simulink model "StandaloneDAQv07_R2014a"  (R2014a)
settings: Solver=FixedStepDiscrete  SolverMode=MultiTasking  StartTime=0.0  StopTime=inf  FixedStep=0.0005  RelTol=1e-3
values from neighbouring files (symbols this model uses):
  ANOMALY_INIT = 10    [DAQParams3_1ms_DDA.m]
  Calibration = getCalibrationParams_ATRIAS()    [DAQParams3_1ms_DDA.m]
  EnableFT = 0    [DAQParams3_1ms_DDA.m]
  EncoderAngleLimits = [60 240; 120 300; 60 240; 120 300; 60 240; 120 300; 60 240; 120 300; -30 30; -30 30; -inf inf; -inf inf; -inf inf; -inf inf; -30 30; -30 30; -inf inf; -90 90; -90 90]*pi/180    [DAQParams3_1ms_DDA.m]
  EncoderFiltSys = getDerivFilter(2, 5, 5, Ts)    [DAQParams3_1ms_DDA.m]
  EncoderThreshold = [5; 5; 5; 5; 5; 5; 5; 5; 5; 5; 250; 250; 250; 250; 5; 5; 5; 5; 5]*pi/180    [DAQParams3_1ms_DDA.m]
  IMUAngleLimits = [-180 180; -90 90; -90 90]*pi/180    [DAQParams3_1ms_DDA.m]
  IMUCommand = 70    [DAQParams3_1ms_DDA.m]
  IMUThreshold = 5*pi/180    (= 0.0872664625997)    [DAQParams3_1ms_DDA.m]
  MAX_ANOMALY = 30    [DAQParams3_1ms_DDA.m]
  MedullaCommand = 0    [DAQParams3_1ms_DDA.m]
  MicrostrainFiltSys = getDerivFilter(2, 5, 5, TsMicrostrain)    [DAQParams3_1ms_DDA.m]
  MODBUS_TIMEOUT = 0.02    [DAQParams3_1ms_DDA.m]
  ResetDAQ = 0    [DAQParams3_1ms_DDA.m]
  ResetYaw = 0    [DAQParams3_1ms_DDA.m]
  STREAMING_TIMEOUT = 0.1    [DAQParams3_1ms_DDA.m]
  TareFT = 0    [DAQParams3_1ms_DDA.m]
  Ts = 0.001    [DAQParams3_1ms_DDA.m]
  UseMicrostrainRate = 0    [DAQParams3_1ms_DDA.m]
undefined symbols (not defined in the file or in its folder): FTCalibration, GearOffset, IMUTorsoOffset, m_XR17D15x, standard
libraries: xpcethercatlib x167, speedgoatlib x13, dspswit3 x2, simulink x2, xpcseriallib x1, SpeedgoatModified x1
(part 3 of 4)

== matlab function StandaloneDAQv07_R2014a/EtherCATNetwork/ComputeEulerAngles ==
  data: RkIn input; wk input; RCal input; Reset input; R0In input; ZYX output; dZYX output; Rk output; R0 output; YawRolloverIn input; YawRollover output
function [ZYX, dZYX, Rk, R0, YawRollover] = fcn(RkIn, wk, RCal, Reset, R0In, YawRolloverIn) %#codegen
    % Convert from IMU frame to robot frame and compute Euler angles. The
    % yaw angle is zeroed whenever (Reset) is true.
        
    if (Reset)
        % Compute the rotation matrix which zeroes the initial yaw
        qT0 = M_to_ZYX(RkIn*RCal);
        R0  = Rz(-qT0(1));
    else
        R0 = R0In;
    end
    
    % Transform from IMU to robot frame and zero initial yaw
    Rk = R0*RkIn*RCal;
    
    % Convert Rk to ZYX Euler angles
    ZYX = M_to_ZYX(Rk);
    
    % Unroll yaw
    YawRolloverCount = YawRolloverIn(1);
    PreviousYaw      = YawRolloverIn(2);
    CurrentYaw       = ZYX(1);
    YawRolloverCount = YawRolloverCount + getYawRollover(CurrentYaw, PreviousYaw);
    YawRollover      = [YawRolloverCount; CurrentYaw];
    ZYX(1)           = ZYX(1) + 2*pi*YawRolloverCount;
    
    % Compute Euler angle derivatives
    qzT = ZYX(1);
    qyT = ZYX(2);
    
    if cos(qyT)>1e-3
        dZYX = [0 -sin(qzT) cos(qzT)*cos(qyT); 0 cos(qzT) sin(qzT)*cos(qyT); 1 0 -sin(qyT)]\(R0*RkIn*wk);
    else
        dZYX = [0; 0; 0];
    end
end

function R = Rz(t)
    R = [cos(t) -sin(t) 0; sin(t) cos(t) 0; 0 0 1];
end

function Rollover = getYawRollover(CurrentYaw, PreviousYaw)
    % Determine if a rollover has occurred on yaw angle If a rollover is
    % detected, the output Rollover is either +1 or -1, depending on the
    % direction of the rollover.
  
    if (PreviousYaw>0 && CurrentYaw < (PreviousYaw-pi))
        Rollover = 1;
    elseif (PreviousYaw<0 && CurrentYaw > (PreviousYaw+pi))
        Rollover = -1;
    else
        Rollover = 0;
    end
end

== matlab function StandaloneDAQv07_R2014a/EtherCATNetwork/EtherCATRobotMicrostrain/ConvertAmpCurrent ==
  data: adc_value input; measuredCurrent output
function measuredCurrent = convert(adc_value)
    %#codegen

    measuredCurrent = (adc_value) * 60.0 / 8192;
end

== matlab function StandaloneDAQv07_R2014a/EtherCATNetwork/EtherCATRobotMicrostrain/ConvertLogicVoltage ==
  data: adc_value input; logicVoltage output
function logicVoltage = convert(adc_value)
    %#codegen
    
    MEDULLA_ADC_MAX_VOLTS     = 2.70;
    MEDULLA_ADC_OFFSET_COUNTS = 172;
    
    logicVoltage = (adc_value - MEDULLA_ADC_OFFSET_COUNTS) * (MEDULLA_ADC_MAX_VOLTS/(4095.0))  * 6.0;
end

== matlab function StandaloneDAQv07_R2014a/EtherCATNetwork/EtherCATRobotMicrostrain/ConvertThermistors ==
  data: Temperatures output; adc_value input
function Temperatures  = convert(adc_value)
    %#codegen
    MEDULLA_ADC_MAX_VOLTS     = 2.70;
    MEDULLA_ADC_OFFSET_COUNTS = 172;
    
    processedADCValue = (adc_value - MEDULLA_ADC_OFFSET_COUNTS) * (MEDULLA_ADC_MAX_VOLTS/(4095.0));
    Temperatures      = (1.0./( (1.0/298.15) + (1.0/3988.0)*log(4700.0./((3.26./processedADCValue) - 1.0)/10000))) - 273.15;
end

== matlab function StandaloneDAQv07_R2014a/StateEstimator/GeneralizedCoordinates ==
  data: EncoderAngles input; EncoderVelocities input; q_clean output; IMUAngles input; IMUVelocities input; UseMotorIncEncoders input; UseIMU input; dq_clean output; IMUTorsoOffset input; GearOffset input; Reset input
function [q_clean, dq_clean] = coords(EncoderAngles, EncoderVelocities, IMUAngles, IMUVelocities, UseMotorIncEncoders, UseIMU, IMUTorsoOffset, GearOffset, Reset)
    %#codegen
    
    % q_clean =
    %  [qzT; qyT; qxT; q1R; q2R; q1L; q2L; qgr1R; qgr2R; q3R; qgr1L; qgr2L; q3L];
    %
    % EncoderAngles = 
    %  [Leg1R; Leg2R; Leg1L; Leg2L; Motor1R; Motor2R; Motor1L; Motor2L; Hip3R; Hip3L; ...   % ABSOLUTE ENCODERS
    %   Inc1R; Inc2R; Inc1L; Inc2L; Inc3R; Inc3L; Boom; Boom; Boom]                         % INCREMENTAL ENCODERS
    
    if (Reset)
        q_clean  = zeros(13,1);
        dq_clean = zeros(13,1);
    else 
        q_clean  = EncoderAngles([17:19 1:6 15 7:8 16]);
        dq_clean = EncoderVelocities([17:19 1:6 15 7:8 16]);
        
        q_clean([8:9 11:12]) = q_clean([8:9 11:12]) + GearOffset*pi/180;
        if (UseMotorIncEncoders)
            if 0
                q_clean([8:9 11:12])  = EncoderAngles(11:14)/50;
                dq_clean([8:9 11:12]) = EncoderVelocities(11:14)/50;
            else
                % BGB 2014-08-29
                % The incremental encoder on q1L was destroyed in the 60V
                % power fault event, so it cannot be used until it is
                % replaced.
                q_clean([8:9 12])  = EncoderAngles([11:12 14])/50;
                dq_clean([8:9 12]) = EncoderVelocities([11:12 14])/50;
            end
        end
        
        if (UseIMU)
            q_clean(1:3)  = IMUAngles + [0; IMUTorsoOffset]*pi/180;
            dq_clean(1:3) = IMUVelocities;
        end
    end
end

== matlab function StandaloneDAQv07_R2014a/EtherCATNetwork/calibrate ==
  data: Calibration input; AbsEncoders input; IncEncoders input; IncEncodersPrev input; AbsAngle output; Reset input; IncAngle output; RolloverIn input; Rollover output; IncCalTickIn input; IncCalTick output
function [AbsAngle, IncAngle, Rollover, IncCalTick] = calibrate(Calibration,AbsEncoders,IncEncoders,IncEncodersPrev,Reset,RolloverIn,IncCalTickIn)
    %#codegen
    [AbsAngle, IncAngle, Rollover, IncCalTick] = calibrateEncoders2(Calibration,AbsEncoders,IncEncoders,IncEncodersPrev,Reset,RolloverIn,IncCalTickIn);
end

== matlab function StandaloneDAQv07_R2014a/EtherCATNetwork/EtherCATRobotMicrostrain/IMU_Medulla/TypecastAndCast ==
  data: u input uint32; y output
function y = unit32_to_double(u)
    %#codegen
    ys = typecast(u, 'single');
    y  = double(ys);
end

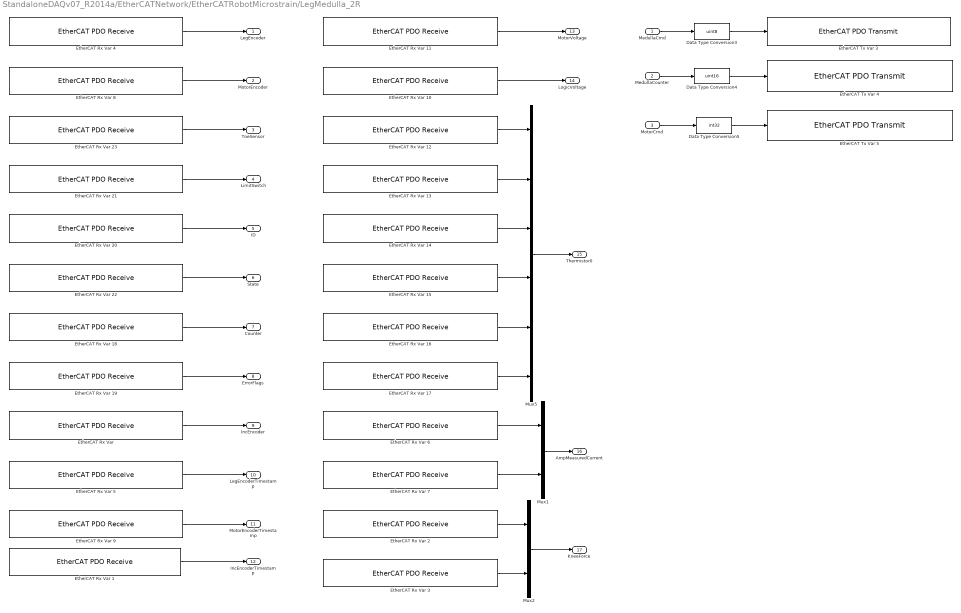
== system StandaloneDAQv07_R2014a/EtherCATNetwork/EtherCATRobotMicrostrain/LegMedulla_2R ==
  MedullaCmd : Inport
  MedullaCounter : Inport  Port=2
  MotorCmd : Inport  Port=3
  Data Type Conversion3 : DataTypeConversion  OutDataTypeStr=uint8  RndMeth=Simplest
  Data Type Conversion4 : DataTypeConversion  OutDataTypeStr=uint16  RndMeth=Simplest
  Data Type Conversion5 : DataTypeConversion  OutDataTypeStr=int32  RndMeth=Simplest
  "EtherCAT Rx Var " : xpcethercatlib/EtherCAT PDO Receive  Priority=2  sig_name=Box 4 (ATRIAS 2.1 Leg (Medulla 1.5)).Incremental Encoder.Incremental Encoder  sig_offset=1872  sig_type=uint16  type_size=16  sig_dim=1  device_id=0  sample_time=0.000500
  EtherCAT Rx Var 1 : xpcethercatlib/EtherCAT PDO Receive  Priority=2  sig_name=Box 4 (ATRIAS 2.1 Leg (Medulla 1.5)).Incremental Encoder.Incremental Encoder Timestamp  sig_offset=1888  sig_type=uint16  type_size=16  sig_dim=1  device_id=0  sample_time=0.000500
  EtherCAT Rx Var 10 : xpcethercatlib/EtherCAT PDO Receive  Priority=2  sig_name=Box 4 (ATRIAS 2.1 Leg (Medulla 1.5)).Power.Logic Voltage  sig_offset=1920  sig_type=uint16  type_size=16  sig_dim=1  device_id=0  sample_time=0.000500
  EtherCAT Rx Var 11 : xpcethercatlib/EtherCAT PDO Receive  Priority=2  sig_name=Box 4 (ATRIAS 2.1 Leg (Medulla 1.5)).Power.Motor Voltage  sig_offset=1904  sig_type=uint16  type_size=16  sig_dim=1  device_id=0  sample_time=0.000500
  EtherCAT Rx Var 12 : xpcethercatlib/EtherCAT PDO Receive  Priority=2  sig_name=Box 4 (ATRIAS 2.1 Leg (Medulla 1.5)).Thermistors.Thermistor 0  sig_offset=1936  sig_type=uint16  type_size=16  sig_dim=1  device_id=0  sample_time=0.000500
  EtherCAT Rx Var 13 : xpcethercatlib/EtherCAT PDO Receive  Priority=2  sig_name=Box 4 (ATRIAS 2.1 Leg (Medulla 1.5)).Thermistors.Thermistor 1  sig_offset=1952  sig_type=uint16  type_size=16  sig_dim=1  device_id=0  sample_time=0.000500
  EtherCAT Rx Var 14 : xpcethercatlib/EtherCAT PDO Receive  Priority=2  sig_name=Box 4 (ATRIAS 2.1 Leg (Medulla 1.5)).Thermistors.Thermistor 2  sig_offset=1968  sig_type=uint16  type_size=16  sig_dim=1  device_id=0  sample_time=0.000500
  EtherCAT Rx Var 15 : xpcethercatlib/EtherCAT PDO Receive  Priority=2  sig_name=Box 4 (ATRIAS 2.1 Leg (Medulla 1.5)).Thermistors.Thermistor 3  sig_offset=1984  sig_type=uint16  type_size=16  sig_dim=1  device_id=0  sample_time=0.000500
  EtherCAT Rx Var 16 : xpcethercatlib/EtherCAT PDO Receive  Priority=2  sig_name=Box 4 (ATRIAS 2.1 Leg (Medulla 1.5)).Thermistors.Thermistor 4  sig_offset=2000  sig_type=uint16  type_size=16  sig_dim=1  device_id=0  sample_time=0.000500
  EtherCAT Rx Var 17 : xpcethercatlib/EtherCAT PDO Receive  Priority=2  sig_name=Box 4 (ATRIAS 2.1 Leg (Medulla 1.5)).Thermistors.Thermistor 5  sig_offset=2016  sig_type=uint16  type_size=16  sig_dim=1  device_id=0  sample_time=0.000500
  EtherCAT Rx Var 18 : xpcethercatlib/EtherCAT PDO Receive  Priority=2  sig_name=Box 4 (ATRIAS 2.1 Leg (Medulla 1.5)).uController Status.Counter  sig_offset=1736  sig_type=uint8  type_size=8  sig_dim=1  device_id=0  sample_time=0.000500
  EtherCAT Rx Var 19 : xpcethercatlib/EtherCAT PDO Receive  Priority=2  sig_name=Box 4 (ATRIAS 2.1 Leg (Medulla 1.5)).uController Status.Error Flags  sig_offset=1744  sig_type=uint8  type_size=8  sig_dim=1  device_id=0  sample_time=0.000500
  EtherCAT Rx Var 2 : xpcethercatlib/EtherCAT PDO Receive  Priority=2  sig_name=Box 4 (ATRIAS 2.1 Leg (Medulla 1.5)).Knee Force.Knee Force 1  sig_offset=2064  sig_type=uint16  type_size=16  sig_dim=1  device_id=0  sample_time=0.000500
  EtherCAT Rx Var 20 : xpcethercatlib/EtherCAT PDO Receive  Priority=2  sig_name=Box 4 (ATRIAS 2.1 Leg (Medulla 1.5)).uController Status.ID  sig_offset=1720  sig_type=uint8  type_size=8  sig_dim=1  device_id=0  sample_time=0.000500
  EtherCAT Rx Var 21 : xpcethercatlib/EtherCAT PDO Receive  Priority=2  sig_name=Box 4 (ATRIAS 2.1 Leg (Medulla 1.5)).uController Status.Limit Switch  sig_offset=1752  sig_type=uint8  type_size=8  sig_dim=1  device_id=0  sample_time=0.000500
  EtherCAT Rx Var 22 : xpcethercatlib/EtherCAT PDO Receive  Priority=2  sig_name=Box 4 (ATRIAS 2.1 Leg (Medulla 1.5)).uController Status.State  sig_offset=1728  sig_type=uint8  type_size=8  sig_dim=1  device_id=0  sample_time=0.000500
  EtherCAT Rx Var 23 : xpcethercatlib/EtherCAT PDO Receive  Priority=2  sig_name=Box 4 (ATRIAS 2.1 Leg (Medulla 1.5)).uController Status.Toe Sensor  sig_offset=1760  sig_type=uint16  type_size=16  sig_dim=1  device_id=0  sample_time=0.000500
  EtherCAT Rx Var 3 : xpcethercatlib/EtherCAT PDO Receive  Priority=2  sig_name=Box 4 (ATRIAS 2.1 Leg (Medulla 1.5)).Knee Force.Knee Force 2  sig_offset=2080  sig_type=uint16  type_size=16  sig_dim=1  device_id=0  sample_time=0.000500
  EtherCAT Rx Var 4 : xpcethercatlib/EtherCAT PDO Receive  Priority=2  sig_name=Box 4 (ATRIAS 2.1 Leg (Medulla 1.5)).Leg Encoder.Leg Encoder  sig_offset=1824  sig_type=uint32  type_size=32  sig_dim=1  device_id=0  sample_time=0.000500
  EtherCAT Rx Var 5 : xpcethercatlib/EtherCAT PDO Receive  Priority=2  sig_name=Box 4 (ATRIAS 2.1 Leg (Medulla 1.5)).Leg Encoder.Leg Encoder Timestamp  sig_offset=1856  sig_type=uint16  type_size=16  sig_dim=1  device_id=0  sample_time=0.000500
  EtherCAT Rx Var 6 : xpcethercatlib/EtherCAT PDO Receive  Priority=2  sig_name=Box 4 (ATRIAS 2.1 Leg (Medulla 1.5)).Measured Current.Amp 1 Measured Current  sig_offset=2032  sig_type=int16  type_size=16  sig_dim=1  device_id=0  sample_time=0.000500
  EtherCAT Rx Var 7 : xpcethercatlib/EtherCAT PDO Receive  Priority=2  sig_name=Box 4 (ATRIAS 2.1 Leg (Medulla 1.5)).Measured Current.Amp 2 Measured Current  sig_offset=2048  sig_type=int16  type_size=16  sig_dim=1  device_id=0  sample_time=0.000500
  EtherCAT Rx Var 8 : xpcethercatlib/EtherCAT PDO Receive  Priority=2  sig_name=Box 4 (ATRIAS 2.1 Leg (Medulla 1.5)).Motor Encoder.Motor Encoder  sig_offset=1776  sig_type=uint32  type_size=32  sig_dim=1  device_id=0  sample_time=0.000500
  EtherCAT Rx Var 9 : xpcethercatlib/EtherCAT PDO Receive  Priority=2  sig_name=Box 4 (ATRIAS 2.1 Leg (Medulla 1.5)).Motor Encoder.Motor Encoder Timestamp  sig_offset=1808  sig_type=uint16  type_size=16  sig_dim=1  device_id=0  sample_time=0.000500
  EtherCAT Tx Var 3 : xpcethercatlib/EtherCAT PDO Transmit   Priority=3  sig_name=Box 4 (ATRIAS 2.1 Leg (Medulla 1.5)).uControllerInput.Command  sig_offset=1720  sig_type=uint8  type_size=8  sig_dim=1  device_id=0  sample_time=0.000500
  EtherCAT Tx Var 4 : xpcethercatlib/EtherCAT PDO Transmit   Priority=3  sig_name=Box 4 (ATRIAS 2.1 Leg (Medulla 1.5)).uControllerInput.Counter  sig_offset=1728  sig_type=uint16  type_size=16  sig_dim=1  device_id=0  sample_time=0.000500
  EtherCAT Tx Var 5 : xpcethercatlib/EtherCAT PDO Transmit   Priority=3  sig_name=Box 4 (ATRIAS 2.1 Leg (Medulla 1.5)).uControllerInput.Motor Current  sig_offset=1744  sig_type=int32  type_size=32  sig_dim=1  device_id=0  sample_time=0.000500
  Mux1 : Mux  Inputs=2
  Mux2 : Mux  Inputs=2
  Mux5 : Mux  Inputs=6
  LegEncoder : Outport
  MotorEncoder : Outport  Port=2
  ToeSensor : Outport  Port=3
  LimitSwitch : Outport  Port=4
  ID : Outport  Port=5
  State : Outport  Port=6
  Counter : Outport  Port=7
  ErrorFlags : Outport  Port=8
  IncEncoder : Outport  Port=9
  LegEncoderTimestamp : Outport  Port=10
  MotorEncoderTimestamp : Outport  Port=11
  IncEncoderTimestamp : Outport  Port=12
  MotorVoltage : Outport  Port=13
  LogicVoltage : Outport  Port=14
  Thermistor0 : Outport  Port=15
  AmpMeasuredCurrent : Outport  Port=16
  KneeForce : Outport  Port=17
  wires:
  Data Type Conversion3/1 -> EtherCAT Tx Var 3/1
  Data Type Conversion4/1 -> EtherCAT Tx Var 4/1
  Data Type Conversion5/1 -> EtherCAT Tx Var 5/1
  "EtherCAT Rx Var "/1 -> IncEncoder/1
  EtherCAT Rx Var 1/1 -> IncEncoderTimestamp/1
  EtherCAT Rx Var 2/1 -> Mux2/1
  EtherCAT Rx Var 3/1 -> Mux2/2
  EtherCAT Rx Var 4/1 -> LegEncoder/1
  EtherCAT Rx Var 5/1 -> LegEncoderTimestamp/1
  EtherCAT Rx Var 6/1 -> Mux1/1
  EtherCAT Rx Var 7/1 -> Mux1/2
  EtherCAT Rx Var 8/1 -> MotorEncoder/1
  EtherCAT Rx Var 9/1 -> MotorEncoderTimestamp/1
  EtherCAT Rx Var 10/1 -> LogicVoltage/1
  EtherCAT Rx Var 11/1 -> MotorVoltage/1
  EtherCAT Rx Var 12/1 -> Mux5/1
  EtherCAT Rx Var 13/1 -> Mux5/2
  EtherCAT Rx Var 14/1 -> Mux5/3
  EtherCAT Rx Var 15/1 -> Mux5/4
  EtherCAT Rx Var 16/1 -> Mux5/5
  EtherCAT Rx Var 17/1 -> Mux5/6
  EtherCAT Rx Var 18/1 -> Counter/1
  EtherCAT Rx Var 19/1 -> ErrorFlags/1
  EtherCAT Rx Var 20/1 -> ID/1
  EtherCAT Rx Var 21/1 -> LimitSwitch/1
  EtherCAT Rx Var 22/1 -> State/1
  EtherCAT Rx Var 23/1 -> ToeSensor/1
  MedullaCmd/1 -> Data Type Conversion3/1
  MedullaCounter/1 -> Data Type Conversion4/1
  MotorCmd/1 -> Data Type Conversion5/1
  Mux5/1 -> Thermistor0/1
  Mux1/1 -> AmpMeasuredCurrent/1
  Mux2/1 -> KneeForce/1

== system StandaloneDAQv07_R2014a/EtherCATNetwork/IMUFilters/CheckAndFilterIMU ==
  q_daq : Inport
  q_limits : Inport  Port=2
  Threshold : Inport  Port=3
  Reset : Inport  Port=4
  IMURate : Inport  Port=5
  UseIMURate : Inport  Port=6
  AnomalyDetection : Stateflow chart  TreatAsAtomicUnit=on  SystemSampleTime=MicrostrainFiltSys.dt
  Constant : Constant  Value=MicrostrainFiltSys.dt
  Discrete State-Space : DiscreteStateSpace  A=MicrostrainFiltSys.A  B=MicrostrainFiltSys.B  C=MicrostrainFiltSys.C  D=MicrostrainFiltSys.D  X0=MicrostrainFiltSys.x0  SampleTime=MicrostrainFiltSys.dt
  Rate Transition{,3..7} (6 alike) : RateTransition  OutPortSampleTimeMultiple=2
  Rate Transition1 : RateTransition  Deterministic=off  OutPortSampleTime=Ts
  Rate Transition2 : RateTransition  Deterministic=off  OutPortSampleTime=Ts
  Rate Transition8 : RateTransition  Deterministic=off  OutPortSampleTime=Ts
  Switch : Switch  Criteria=u2 ~= 0  Threshold=0.5
  Unit Delay : UnitDelay  SampleTime=MicrostrainFiltSys.dt
  q_clean : Outport
  dq_clean : Outport  Port=2
  ErrorCount : Outport  Port=3
  wires:
  Unit Delay/1 -> AnomalyDetection/2(dq)
  Threshold/1 -> Rate Transition5/1
  q_daq/1 -> Rate Transition/1
  AnomalyDetection/1(q_clean) -> Rate Transition1/1, Discrete State-Space/1
  Rate Transition/1 -> AnomalyDetection/1(q)
  Rate Transition1/1 -> q_clean/1
  Rate Transition2/1 -> dq_clean/1
  Switch/1 -> Rate Transition2/1, Unit Delay/1
  Discrete State-Space/1 -> Switch/3
  IMURate/1 -> Rate Transition3/1
  UseIMURate/1 -> Rate Transition4/1
  Constant/1 -> AnomalyDetection/6(ANOMALY_DT)
  Rate Transition3/1 -> Switch/1
  Rate Transition4/1 -> Switch/2
  Rate Transition5/1 -> AnomalyDetection/4(Threshold)
  q_limits/1 -> Rate Transition6/1
  Reset/1 -> Rate Transition7/1
  Rate Transition6/1 -> AnomalyDetection/3(q_limits)
  Rate Transition7/1 -> AnomalyDetection/5(Reset)
  AnomalyDetection/2(ErrorCount) -> Rate Transition8/1
  Rate Transition8/1 -> ErrorCount/1

== system StandaloneDAQv07_R2014a/SerialInterfaces/FTInterface/ATI Serial NoInt ==
  TX1 : Inport
  TX2 : Inport  Port=2
  Board Setup : speedgoatlib/IO503/Speedgoat IO503 Internal blocks/Board Setup  irqnum=5  slot=slot
  Constant : Constant  OutDataTypeStr=Inherit: Inherit via back propagation  SampleTime=-1
  Constant1 : Constant  OutDataTypeStr=Inherit: Inherit via back propagation  SampleTime=-1
  Count : Selector  IndexMode=Zero-based  Indices=0
  Count1 : Selector  IndexMode=Zero-based  Indices=0
  Read HW FIFO : speedgoatlib/IO503/Speedgoat IO503 Internal blocks/Read HW FIFO  port=1  flush=off  slot=slot
  Read HW FIFO1 : speedgoatlib/IO503/Speedgoat IO503 Internal blocks/Read HW FIFO  port=2  flush=off  slot=slot
  Setup 2 : speedgoatlib/IO503/Speedgoat IO503 Internal blocks/Setup  port=2  transceiver=RS485 half-duplex  standard=on  baudrate=1382400  bauddivisor=1  mode8x=16x (standard)  prescale=off  width=8  nstop=1  parity=Even  rlevel=almost full (56)  ctsmode=none  xonoff=none  xon=17  xoff=19  rs485mode=on  rs485delay=0  slot=slot
  "Setup1 " : speedgoatlib/IO503/Speedgoat IO503 Internal blocks/Setup  port=1  transceiver=RS485 half-duplex  standard=on  baudrate=1382400  bauddivisor=1  mode8x=16x (standard)  prescale=off  width=8  nstop=1  parity=Even  rlevel=almost full (56)  ctsmode=none  xonoff=none  xon=17  xoff=19  rs485mode=on  rs485delay=0  slot=slot
  Write HW FIFO : speedgoatlib/IO503/Speedgoat IO503 Internal blocks/Write HW FIFO  port=1  slot=slot
  Write HW FIFO1 : speedgoatlib/IO503/Speedgoat IO503 Internal blocks/Write HW FIFO  port=2  slot=slot
  RX1 : Outport  SourceOfInitialOutputValue=Input signal
  RX2 : Outport  Port=2  SourceOfInitialOutputValue=Input signal
  wires:
  Read HW FIFO/1 -> RX1/1
  Constant/1 -> Read HW FIFO/1
  Read HW FIFO1/1 -> RX2/1
  Constant1/1 -> Read HW FIFO1/1
  Count/1 -> Write HW FIFO/2
  Count1/1 -> Write HW FIFO1/2
  TX1/1 -> Count/1, Write HW FIFO/1
  TX2/1 -> Count1/1, Write HW FIFO1/1

== system StandaloneDAQv07_R2014a/SerialInterfaces/FTInterface/Subsystem ==
  CalibrationSet : Inport  Partition=off
  Tare : Inport  Port=2  Partition=off
  Reset : Inport  Port=3  Partition=off
  SerialIn : Inport  Port=4  Partition=on  PartitionDimension=1  PartitionWidth=65
  ComputeCalibratedTorques : Subsystem
  FTStateMachine : Stateflow chart  TreatAsAtomicUnit=on
  For Each : ForEach  DisableCoverage=on  IndexMode=One-based
  FTStatus : Outport  ConcatenationDimension=1
  FT : Outport  Port=2  ConcatenationDimension=1
  FTInterfaceStatus : Outport  Port=3  ConcatenationDimension=1
  FTSetupStatus : Outport  Port=4  ConcatenationDimension=1
  CalibrationSerial : Outport  Port=5  ConcatenationDimension=1
  SerialOut : Outport  Port=6  ConcatenationDimension=1
  wires:
  SerialIn/1 -> FTStateMachine/3(SerialIn)
  FTStateMachine/4(FTInterfaceStatus) -> FTInterfaceStatus/1
  FTStateMachine/6(SerialOut) -> SerialOut/1
  CalibrationSet/1 -> FTStateMachine/1(CalibrationSet)
  FTStateMachine/5(FTSetupStatus) -> FTSetupStatus/1
  ComputeCalibratedTorques/1(FT) -> FT/1
  FTStateMachine/3(Calibration) -> ComputeCalibratedTorques/2(Cal)
  FTStateMachine/1(GaugeStatus) -> FTStatus/1
  Tare/1 -> ComputeCalibratedTorques/3(Tare)
  Reset/1 -> FTStateMachine/2(Reset)
  FTStateMachine/2(Gauge) -> ComputeCalibratedTorques/1(Gauge)

== system StandaloneDAQv07_R2014a/SerialInterfaces/KVH/Send Receive1 ==
  Board Setup : speedgoatlib/IO503/Speedgoat IO503 Internal blocks/Board Setup  irqnum=9  slot=slot
  Constant : Constant
  Read HW FIFO : speedgoatlib/IO503/Speedgoat IO503 Internal blocks/Read HW FIFO  port=1  flush=on  slot=slot
  Setup3 : speedgoatlib/IO503/Speedgoat IO503 Internal blocks/Setup  port=3  transceiver=RS422  standard=on  baudrate=921600  bauddivisor=1  mode8x=16x (standard)  prescale=off  width=8  nstop=1  parity=None  rlevel=half full (32)  ctsmode=none  xonoff=none  xon=17  xoff=19  rs485mode=off  rs485delay=0  slot=slot
  Rx3 : Outport
  wires:
  Read HW FIFO/1 -> Rx3/1
  Constant/1 -> Read HW FIFO/1

== system StandaloneDAQv07_R2014a/SerialInterfaces/KVH/Subsystem ==
  Board Setup : speedgoatlib/IO503/Speedgoat IO503 Internal blocks/Board Setup  irqnum=9  slot=slot
  Constant : Constant  OutDataTypeStr=uint32  SampleTime=-1
  FIFO write 1 : xpcseriallib/FIFO write   size=256  inputtype=count+32 bit uint  present=off  sampletime=-1  id=IO503: KVH Interface
  Read HW FIFO : speedgoatlib/IO503/Speedgoat IO503 Internal blocks/Read HW FIFO  port=3  flush=on  slot=slot
  Setup3 : speedgoatlib/IO503/Speedgoat IO503 Internal blocks/Setup  port=3  transceiver=RS422  standard=on  baudrate=921600  bauddivisor=1  mode8x=16x (standard)  prescale=off  width=8  nstop=1  parity=None  rlevel=almost full (56)  ctsmode=none  xonoff=none  xon=17  xoff=19  rs485mode=off  rs485delay=0  slot=slot
  SerialData : Outport
  wires:
  Constant/1 -> Read HW FIFO/1
  Read HW FIFO/1 -> FIFO write 1/1
  FIFO write 1/1 -> SerialData/1

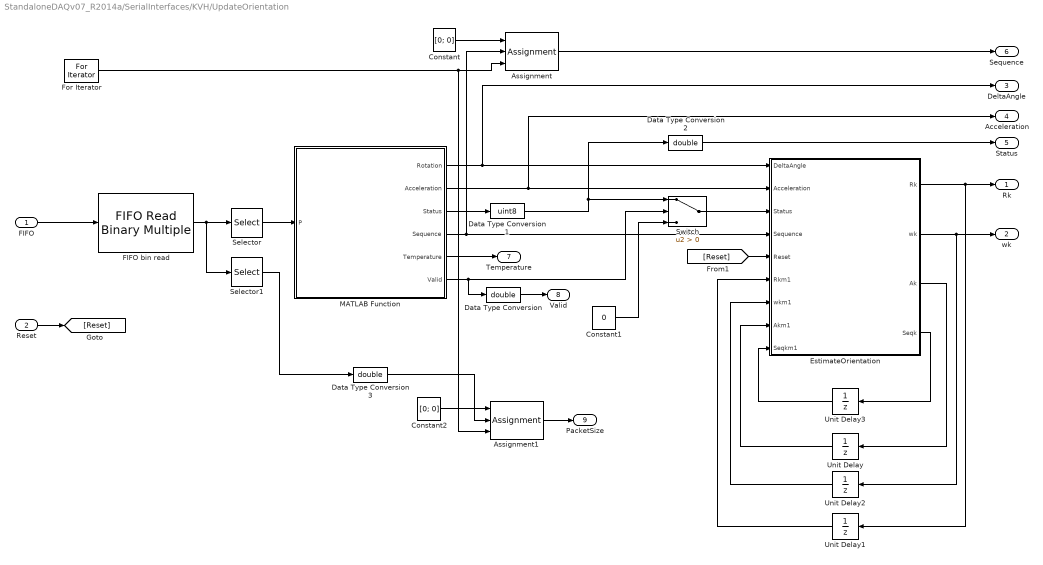
== system StandaloneDAQv07_R2014a/SerialInterfaces/KVH/UpdateOrientation ==
  FIFO : Inport
  Reset : Inport  Port=2
  Assignment : Assignment  IndexMode=Zero-based  IndexOptions=Index vector (port)
  Assignment1 : Assignment  IndexMode=Zero-based  IndexOptions=Index vector (port)
  Constant : Constant  Value=[0; 0]
  Constant1 : Constant  Value=0  OutDataTypeStr=uint8
  Constant2 : Constant  Value=[0; 0]
  Data Type Conversion : DataTypeConversion  OutDataTypeStr=double
  Data Type Conversion1 : DataTypeConversion  OutDataTypeStr=uint8  RndMeth=Simplest
  Data Type Conversion2 : DataTypeConversion  OutDataTypeStr=double
  Data Type Conversion3 : DataTypeConversion  OutDataTypeStr=double
  EstimateOrientation : MATLAB Function  TreatAsAtomicUnit=on
  "FIFO bin read " : SpeedgoatModified/FIFO Read Binary Multiple  header={char([254, 129, 255, 85])}  lengths=36  hold=Zero output if no new data  enable=off  maxsize=36  outputtype=count+32 bit uint  sampletime=-1
  For Iterator : ForIterator  IterationLimit=2  IndexMode=Zero-based
  MATLAB Function : MATLAB Function  TreatAsAtomicUnit=on
  Selector : Selector  IndexMode=Zero-based  InputPortWidth=37  Indices=1:36
  Selector1 : Selector  IndexMode=Zero-based  InputPortWidth=37  Indices=0
  Switch : Switch  Criteria=u2 > Threshold
  Unit Delay : UnitDelay  InitialCondition=[0; 0; 0]  SampleTime=-1
  Unit Delay1 : UnitDelay  InitialCondition=zeros(3,3)  SampleTime=-1
  Unit Delay2 : UnitDelay  InitialCondition=[0; 0; 0]  SampleTime=-1
  Unit Delay3 : UnitDelay  SampleTime=-1
  Rk : Outport  InitialOutput=zeros(3,3)
  wk : Outport  Port=2  InitialOutput=zeros(3,1)
  DeltaAngle : Outport  Port=3  InitialOutput=zeros(3,1)
  Acceleration : Outport  Port=4  InitialOutput=zeros(3,1)
  Status : Outport  Port=5  InitialOutput=0
  Sequence : Outport  Port=6  InitialOutput=[0; 0]
  Temperature : Outport  Port=7  InitialOutput=0
  Valid : Outport  Port=8  InitialOutput=0
  PacketSize : Outport  Port=9  InitialOutput=0
  wires:
  MATLAB Function/2(Acceleration) -> Acceleration/1, EstimateOrientation/2(Acceleration)
  MATLAB Function/1(Rotation) -> DeltaAngle/1, EstimateOrientation/1(DeltaAngle)
  MATLAB Function/3(Status) -> Data Type Conversion1/1
  MATLAB Function/5(Temperature) -> Temperature/1
  EstimateOrientation/3(Ak) -> Unit Delay/1
  Unit Delay/1 -> EstimateOrientation/8(Akm1)
  EstimateOrientation/1(Rk) -> Rk/1, Unit Delay1/1
  Unit Delay1/1 -> EstimateOrientation/6(Rkm1)
  [Reset] -> EstimateOrientation/5(Reset)
  Switch/1 -> EstimateOrientation/3(Status)
  MATLAB Function/6(Valid) -> Switch/2, Data Type Conversion/1
  EstimateOrientation/4(Seqk) -> Unit Delay3/1
  Unit Delay3/1 -> EstimateOrientation/9(Seqkm1)
  Reset/1 -> [Reset]
  FIFO/1 -> "FIFO bin read "/1
  EstimateOrientation/2(wk) -> wk/1, Unit Delay2/1
  Unit Delay2/1 -> EstimateOrientation/7(wkm1)
  "FIFO bin read "/1 -> Selector1/1, Selector/1
  MATLAB Function/4(Sequence) -> EstimateOrientation/4(Sequence), Assignment/2
  Assignment/1 -> Sequence/1
  Constant/1 -> Assignment/1
  Selector/1 -> MATLAB Function/1(P)
  Data Type Conversion/1 -> Valid/1
  Data Type Conversion1/1 -> Data Type Conversion2/1, Switch/1
  Constant1/1 -> Switch/3
  Data Type Conversion2/1 -> Status/1
  Selector1/1 -> Data Type Conversion3/1
  Constant2/1 -> Assignment1/1
  For Iterator/1 -> Assignment1/3, Assignment/3
  Assignment1/1 -> PacketSize/1
  Data Type Conversion3/1 -> Assignment1/2

== system StandaloneDAQv07_R2014a/SerialInterfaces/FTInterface/Subsystem/ComputeCalibratedTorques ==
  Gauge : Inport
  Cal : Inport  Port=2
  Tare : Inport  Port=3
  ComputeCalibratedTorques : MATLAB Function  TreatAsAtomicUnit=on
  Latch : Subsystem
  Reshape : Reshape
  FT : Outport
  wires:
  Gauge/1 -> Latch/1(Gauge), ComputeCalibratedTorques/1(Gauge)
  ComputeCalibratedTorques/1(FT) -> Reshape/1
  Cal/1 -> ComputeCalibratedTorques/3(Cal)
  Tare/1 -> Latch/Enable
  Reshape/1 -> FT/1
  Latch/1(Bias) -> ComputeCalibratedTorques/2(Bias)

== system StandaloneDAQv07_R2014a/SerialInterfaces/FTInterface/Subsystem/ComputeCalibratedTorques/Latch ==
  Gauge : Inport
  Tare : EnablePort
  Bias : Outport  InitialOutput=zeros(6,1,'uint16')
  wires:
  Gauge/1 -> Bias/1

== stateflow chart StandaloneDAQv07_R2014a/EtherCATNetwork/IMUFilters/CheckAndFilterIMU/AnomalyDetection ==
  state Run
    state Nominal
      en, du:
      q_clean = q;
      q_last = q;
      dq_last = dq;
      ErrorCount = 0;
    state Error
      en: dq_last = dq; //dq is delayed to prevent algebraic loops
      en, du:
      ErrorCount++;
      q_clean = q_last + ErrorCount*dq_last*ANOMALY_DT;
    (default) -> Nominal
    Nominal -> Error : [check_error()]
    Error -> Nominal [order 2] : [!check_error()]
  state Init
    en, du:
    q_clean = q;
    q_last = q;
    dq_last = dq;
    ErrorCount = 0;
  (default) -> Init
  Init -> Run : [!Reset && after(ANOMALY_INIT, tick)]
  Run -> Init : [Reset]
  Error -> Init [order 1] : [ErrorCount>MAX_ANOMALY]
  data: err function_output boolean; q input size=1; dq input size=1; q_clean output double size=1; ErrorCount output double; MAX_ANOMALY parameter double size=1; q_last local double size=1; dq_last local double size=1; ANOMALY_INIT parameter double size=1; q_limits input double size=2; Threshold input size=1; Reset input boolean size=1; ANOMALY_DT input double size=1
  function err = check_error:
    | function err = check_error
    |     %#codegen
    |     err = (q<q_limits(1)) || (q>q_limits(2)) || (abs(q - q_clean) > (ErrorCount+1)*Threshold); 
    | end

== matlab function StandaloneDAQv07_R2014a/EtherCATNetwork/EtherCATRobotMicrostrain/IMU_Medulla/TypecastAndCast1 ==
  data: u input uint32; y output
function y = unit32_to_double(u)
    %#codegen
    ys = typecast(u, 'single');
    y  = double(ys);
end

== stateflow chart StandaloneDAQv07_R2014a/SerialInterfaces/FTInterface/Subsystem/FTStateMachine ==
  state Run
    state FTSetup [parallel]
      settings: executionOrder=1
      state ModbusMode
        entry:
        clearModbusCommand();
        clearCalibration();
        RequestStreamingMode = 0;
        state SetSessionId
          entry:
          FTSetupStatus = 2;
        state ReadCalibration
          entry:
          clearCalibration();
          state SendRequest
            entry:
            FTSetupStatus = 3;
            requestCalibration();
            during:
            clearModbusCommand();
          state ParseRequest
            entry:
            FTSetupStatus = 4;
            parseCalibration();
          (default) -> SendRequest
          SendRequest -> ParseRequest [order 1] : [validResponse()]
          ParseRequest -> SendRequest [order 1] : [CalibrationBufferEnd<338]
          SendRequest -> SendRequest [order 2] : [after(0.2,sec)]
        state WriteActiveCalibration
          entry:
          FTSetupStatus = 1.30;
          (history)
          state LockStorage
            entry:
            FTSetupStatus = 8;
            lockUnlockStorage(0);
            during:
            clearModbusCommand();
          state writeActiveCal
            entry:
            FTSetupStatus = 7;
            writeActiveCalibration();
            during:
            clearModbusCommand();
          state readActiveCal
            entry:
            FTSetupStatus = 5;
            readActiveCalibration();
            during:
            clearModbusCommand();
          state UnlockStorage
            entry:
            FTSetupStatus = 6;
            lockUnlockStorage(1);
            during:
            clearModbusCommand();
          (default) -> readActiveCal
          writeActiveCal -> LockStorage : [validResponse()]
          LockStorage -> readActiveCal : [validResponse()]
          UnlockStorage -> writeActiveCal : [validResponse()]
          readActiveCal -> UnlockStorage [order 2] : [validResponse()]
        (default) -> SetSessionId
        SetSessionId -> ReadCalibration
        ParseRequest -> WriteActiveCalibration [order 2]
        WriteActiveCalibration -> WriteActiveCalibration : [after(2*MODBUS_TIMEOUT, sec)]
      state Initialize
        entry:
        FTSetupStatus = 0;
        clearModbusCommand();
        clearCalibration();
        RequestStreamingMode = 0;
      state StreamingMode
        entry:
        FTSetupStatus = 9;
        clearModbusCommand();
        RequestStreamingMode = 1;
      (default) -> Initialize
      Initialize -> Run.FTSetup.ModbusMode : [FTInterfaceStatus == 5]
      readActiveCal -> Run.FTSetup.StreamingMode [order 1] : [validResponse() && verifyActiveCalibration()]
    state FTInterface [parallel]
      settings: executionOrder=2
      state ModbusMode
        entry:
        clearGauge();
        clearSerialOut();
        state ModbusIdle
          entry:
          FTInterfaceStatus = 5;
          clearModbusResponse();
          clearSerialBuffer();
        state ModbusSend
          entry:
          FTInterfaceStatus = 6;
          clearSerialBuffer();
          sendModbusCmd(ModbusCommand);
          exit:
          clearSerialOut();
        state ModbusReceive
          entry, during:
          FTInterfaceStatus = 7;
          readModbusResponse()
        state ModbusValidate
          entry:
          FTInterfaceStatus = 8;
          validateModbusResponse();
          exit:
          clearModbusResponse();
        (default) -> ModbusIdle
        (junction 37) -> ModbusIdle
        (junction 99) -> (junction 37) [order 2]
        ModbusIdle -> ModbusSend [order 2] : [ModbusCommand(1)>0]
        (junction 99) -> ModbusSend [order 1] : [ModbusCommand(1)>0]
        (junction 36) -> (junction 99)
        ModbusSend -> ModbusReceive
        ModbusReceive -> (junction 36) [order 2] : [after(MODBUS_TIMEOUT, sec)]
        (junction 86) -> (junction 36)
        ModbusReceive -> ModbusValidate [order 1] : [Valid]
        ModbusValidate -> (junction 86)
      state InitializeStreaming
        entry:
        FTInterfaceStatus = 3;
        clearSerialBuffer();
        sendStreamingCmd(1);
        exit:
        clearSerialOut();
      state CheckStreaming
        state WaitClear
          entry:
          FTInterfaceStatus = 1;
          clearSerialOut();
          clearSerialBuffer();
        state CheckSerialInput
          entry:
          FTInterfaceStatus = 2;
        (default) -> WaitClear
        WaitClear -> CheckSerialInput
      state StreamingMode
        entry:
        FTInterfaceStatus = 9;
        clearGauge();
        clearSerialOut();
        clearSerialBuffer();
        during:
        parseStreamingData();
      state EndStreaming
        entry:
        FTInterfaceStatus = 4;
        clearSerialBuffer();
        sendStreamingCmd(0);
        exit:
        clearSerialOut();
      ModbusIdle -> InitializeStreaming [order 1] : [RequestStreamingMode ~= 0]
      InitializeStreaming -> CheckStreaming
      (default) -> CheckStreaming
      CheckSerialInput -> Run.FTInterface.ModbusMode [order 2] : [after(STREAMING_TIMEOUT, sec)]
      CheckSerialInput -> Run.FTInterface.StreamingMode [order 1] : [SerialIn(1)>0]
      EndStreaming -> CheckStreaming
      Run.FTInterface.StreamingMode -> EndStreaming : [RequestStreamingMode==0]
  state Reset
    entry:
    FTSetupStatus = 0;
    FTInterfaceStatus = 0;
    clearModbusCommand();
    clearModbusResponse();
    clearCalibration();
    clearGauge();
    clearSerialBuffer();
    clearSerialOut();
  (default) -> Reset
  Reset -> Run : [Reset==0]
  Run -> Reset : [Reset>0]
  data: valid function_output; Unlock function_input; ok function_output; Command function_input; Select function_input; CalibrationSet input; Reset input; RequestStreamingMode local; SerialBuffer local; SerialBufferEnd local; GaugeStatus output; Gauge output; Calibration output Bus: FTCalibrationBus; ModbusCommand local; ModbusResponse local; FTInterfaceStatus output; SerialIn input; ResponseLength local; LastModbusFunction local; MODBUS_TIMEOUT parameter; STREAMING_TIMEOUT parameter; Valid local; FTSetupStatus output; SerialOut output; FTCalibration parameter Bus: FTCalibrationBus; CalibrationBuffer local; CalibrationBufferEnd local
  function requestCalibration:
    | function requestCalibration() %#codegen
    |    % ATI F/T Calibration data are stored in 16-bit holding registers. There
    |    % are 16 calibration sets, each 338 bytes (or 169 registers) long. They
    |    % are stored beginning at holding register address 0x00e3 (Calibration
    |    % 1). Subsequent calibration sets are spaced 192 holding registers
    |    % apart.
    |    BaseAddress = uint32(hex2dec('00e3')) + uint32(192 * (CalibrationSet - 1));
    |    
    |    % Calibration data must be read in two or more parts due to length
    |    % restricitons in the Modbus protocol. In order to keep buffer sizes
    |    % small we'll read in parts of no more than 12 registers each.
    |    
    |    NextCalibrationRegister = uint32(CalibrationBufferEnd/2);
    |    Address = BaseAddress + NextCalibrationRegister;
    |    NumRegs = min(12, 169 - NextCalibrationRegister);
    |    
    |    ModbusFunction = 3;
    |    ModbusCommand(1:6) = uint32([5; ModbusFunction; bitshift(Address,-8); bitand(Address,255); 0; NumRegs]);
    | end
  function parseCalibration:
    | function parseCalibration() %#codegen
    |     % Calibration data must be read in two or more parts due to length
    |     % restricitons in the Modbus protocol.
    |     
    |     NumBytes = min(ModbusResponse(3), length(CalibrationBuffer) - CalibrationBufferEnd);
    |     CalibrationBuffer(CalibrationBufferEnd+(1:NumBytes)) = ModbusResponse(3+(1:NumBytes));
    |     CalibrationBufferEnd = CalibrationBufferEnd + NumBytes;
    |     if (CalibrationBufferEnd==338)
    |         Calibration = parseFTCalibration2(CalibrationBuffer(1:CalibrationBufferEnd));
    |     end
    | end
    | 
    | function Cal = parseFTCalibration2(CalibrationBuffer)
    |     Cal.CalibSerialNumber = parseUint8(CalibrationBuffer(1:8));
    |     Cal.CalibPartNumber   = parseUint8(CalibrationBuffer(9:40));
    |     Cal.CalibFamilyId     = parseUint8(CalibrationBuffer(41:44));
    |     Cal.CalibTime         = parseUint8(CalibrationBuffer(45:64));
    |     Cal.BasicMatrix       = reshape(parseFloat(CalibrationBuffer(65:208)), 6, 6).';
    |     Cal.ForceUnits        = parseUint8(CalibrationBuffer(209));
    |     Cal.TorqueUnits       = parseUint8(CalibrationBuffer(210));
    |     Cal.MaxRating         = parseFloat(CalibrationBuffer(211:234));
    |     Cal.CountsPerForce    = parseInt32(CalibrationBuffer(235:238));
    |     Cal.CountsPerTorque   = parseInt32(CalibrationBuffer(239:242));
    |     Cal.GageGain          = parseUint16(CalibrationBuffer(243:254));
    |     Cal.GageOffset        = parseUint16(CalibrationBuffer(255:266));
    |     Cal.Resolution        = parseUint8(CalibrationBuffer(267:272));
    |     Cal.Range             = parseUint8(CalibrationBuffer(273:278));
    |     Cal.ScaleFactor16     = parseUint16(CalibrationBuffer(279:290));
    |     Cal.UserField1        = parseUint8(CalibrationBuffer(291:306));
    |     Cal.UserField2        = parseUint8(CalibrationBuffer(307:322));
    |     Cal.SpareData         = parseUint8(CalibrationBuffer(323:338));
    | end
    | 
    | 
    | function d = parseUint8(D)
    |     d = double(D);
    | end
    | 
    | function d = parseFloat(D)
    |     D1 = uint32(D);
    |     D2 = bitshift(D1(1:4:end), 24) + bitshift(D1(2:4:end), 16) + bitshift(D1(3:4:end), 8) + D1(4:4:end);
    |     d = double(typecast(D2, 'single'));
    | end
    | 
    | function d = parseUint32(D)
    |     D1 = uint32(D);
    |     D2 = bitshift(D1(1:4:end), 24) + bitshift(D1(2:4:end), 16) + bitshift(D1(3:4:end), 8) + D1(4:4:end);
    |     d  = double(D2);
    | end
    | 
    | function d = parseInt32(D)
    |     D1 = int32(D);
    |     D2 = bitshift(D1(1:4:end), 24) + bitshift(D1(2:4:end), 16) + bitshift(D1(3:4:end), 8) + D1(4:4:end);
    |     d  = double(D2);
    | end
    | 
    | function d = parseUint16(D)
    |     D1 = uint16(D);
    |     D2 = bitshift(D1(1:2:end), 8) + D1(2:2:end);
    |     d  = double(D2);
    | end
  function valid = validResponse:
    | function valid = validResponse %#codegen
    |     valid = false;
    |     
    |     ModbusFunction = double(ModbusResponse(2));
    |     
    |     if (ModbusResponse(1) > 1)    
    |         switch ModbusFunction
    |             case {3, 6, 16}
    |                 % 3: Read holding registers
    |                 % 6: Write single register
    |                 % 16: Write multiple registers
    |                 
    |                 % If there were an error, the response ModbusFunction code
    |                 % would be (F + 0x80
    |                 valid = true;
    |                 
    |             case {70, 106}
    |                 ModbusByteCount = double(ModbusResponse(3));
    |                 valid = (ModbusByteCount == 1);
    |         end
    |     end
    | end
  function lockUnlockStorage(Unlock):
    | function lockUnlockStorage(Unlock) %#codegen
    |     % ATI F/T Calibration data are stored in holding registers. After
    |     % reading a calibration data set, we must write the GaugeGain and
    |     % GaugeOffset values to the active gain and offset holding registers.
    |     % Before writing to the active gain/offset registers, we must unlock
    |     % the storage.
    |     
    |     ModbusFunction = 106; % Read holding registers
    |     if (Unlock==1)
    |         Data = 170; % hex2dec('aa')
    |     else
    |         Data = 24; % hex2dec('18')
    |     end
    |         
    |     ModbusCommand(1:3) = uint32([2; ModbusFunction; Data]);
    | end
  function readActiveCalibration:
    | function readActiveCalibration %#codegen
    |     % ATI F/T Calibration data are stored in holding registers. After
    |     % reading a calibration data set, we must write the GaugeGain and
    |     % GaugeOffset values to the active gain and offset holding registers.
    |     % Holding register addresses:
    |     %   0x0000-0x0005 Active Gain pots
    |     %   0x0006-0x000B Active Offset DACs
    |     ModbusFunction = 3; % Read holding registers
    |     Address = uint32(0);
    |     NumRegs = 12;
    |     ModbusCommand(1:6) = uint32([5; ModbusFunction; bitshift(Address,-8); bitand(Address,255); 0; NumRegs]);
    | end
  function ok = verifyActiveCalibration:
    | function ok = verifyActiveCalibration %#codegen
    |     % ATI F/T Calibration data are stored in holding registers. After
    |     % reading a calibration data set, we must write the GaugeGain and
    |     % GaugeOffset values to the active gain and offset holding registers.
    |     % Holding register addresses:
    |     %   0x0000-0x0005 Active Gain pots
    |     %   0x0006-0x000B Active Offset DACs
    |     ok = false;
    |     
    |     % Check response length
    |     ActualResponseLength = double(ModbusResponse(1));
    |     if (ActualResponseLength ~= 26)
    |         return
    |     end
    |     
    |     % Compare gain and offset values with those in the calibration
    |     % structure
    |     ActiveGaugeGain   = parseUint16(ModbusResponse(3  + (1:12)));
    |     ActiveGaugeOffset = parseUint16(ModbusResponse(15 + (1:12)));
    |     
    |     if any(ActiveGaugeGain ~= Calibration.GageGain) ...
    |             || any(ActiveGaugeOffset ~= Calibration.GageOffset)
    |         return;
    |     end
    |     
    |     % Then it looks okay
    |     ok = true;
    | end
    | 
    | function u = parseUint16(D)
    |     D1 = double(D);
    |     u = D1(1:2:end)*256 + D1(2:2:end);
    | end
  function writeActiveCalibration:
    | function writeActiveCalibration %#codegen
    |     % ATI F/T Calibration data are stored in holding registers. After
    |     % reading a calibration data set, we must write the GaugeGain and
    |     % GaugeOffset values to the active gain and offset holding registers.
    |     % Holding register addresses:
    |     %   0x0000-0x0005 Active Gain pots
    |     %   0x0006-0x000B Active Offset DACs
    |     ModbusFunction = 16; % Write multiple registers
    |     Address = uint32(0);
    |     NumRegs = 12;
    |     
    |     ModbusCommand(1:31) = uint32([30; ModbusFunction; bitshift(Address,-8); bitand(Address,255); 0; NumRegs; 2*NumRegs; zeros(2*NumRegs, 1, 'uint32')]);
    |     
    |     Data = uint32([Calibration.GageGain Calibration.GageOffset]);
    |     for k=1:NumRegs
    |         ModbusCommand(8 + 2*(k-1)) = bitshift(Data(k), -8); 
    |         ModbusCommand(9 + 2*(k-1)) = bitand(Data(k), 255);
    |     end
    | end
  function parseStreamingData:
    | function parseStreamingData %#codegen
    |     % Look for the last good F/T packet in the SerialIn buffer.
    |     % See section 9.4.2 of 9620-05-Digital FT______________Last_version_300414.pdf at
    |     % https://sites.google.com/a/umich.edu/atrias/knowledge-base/hardware/load-cells
    |     %
    |     % GaugeStatus is a scalar:
    |     %   GaugeStatus = -1   if no valid packets found (no valid checksum)
    |     %   GaugeStatus = 1    if a valid packet was found but the gauge status
    |     %                      bit was set (indicates a strain gauge error)
    |     %   GaugeStatus = 0    if a good packet was found
    |     
    |     Gauge = zeros(6,1);
    |     GaugeStatus = -1;
    |     
    |     numNewBytes = min(SerialIn(1), length(SerialIn)-1);
    |     k = 1;
    |     while (k + 13 <= numNewBytes)
    |         % Verify checksum (first seven bits of last byte in packet)
    |         valid = CheckSample(SerialIn(k+(1:13)));
    |         
    |         if valid
    |             % Get gauge status bit (msb of last byte in packet) if the packet is valid
    |             StatusBit = double(bitget(SerialIn(k+13), 8));
    |             if (StatusBit == 0) || (GaugeStatus == -1)
    |                 Gauge     = ComputeGauge(SerialIn(k+(1:12)));
    |                 GaugeStatus = StatusBit;
    |             end
    |             k = k + 13;
    |         else
    |             k = k + 1;
    |         end 
    |     end
    | end
    | 
    | function valid = CheckSample( sampleBytes )
    |     checkSum = sum(int16(sampleBytes(1:12)), 'native');
    |     valid = bitand(checkSum, 127) == bitand(sampleBytes(13), 127);
    | end
    | 
    | function Gauge = ComputeGauge(D)
    |     % Convert uint8 to int16 and reorder
    |     % The Digital F/T board returns Gauge data in the order
    |     %   [G0 G2 G4 G1 G3 G5]'.
    |     % and we want it in the order
    |     %   [G0 G1 G2 G3 G4 G5].'
    |     
    |     Gauge = double( bitshift(int16(D([1 3 5 7 9 11])), 8) + int16(D([2 4 6 8 10 12])) );
    |     Gauge = Gauge([1 4 2 5 3 6]);
    | end
  function sendModbusCmd(Command):
    | function sendModbusCmd(Command) %#codegen
    |     
    |     % All ATI Digital F/T interface boards use Modbus address 10.
    |     % See ATI Digital F/T System Installation and Operation Manual
    |     % (Document #9620-05-Digital FT).
    |     L = Command(1);
    |     assert(L < 65);
    |     
    |     ModbusAddress  = uint32(10);
    |     ModbusFunction = Command(2);
    |     ModbusData     = Command(1+(2:L));
    |     ModbusPacket   = createModbusPacket32(ModbusAddress, ModbusFunction, ModbusData);
    |     
    |     L = length(ModbusPacket);
    |     SerialOut(1)     = uint32(L);
    |     SerialOut(2:L+1) = ModbusPacket;
    |     
    |     % Expected response length
    |     ResponseLength = getModbusResponseLength32(ModbusFunction, ModbusData);
    |     
    |     % Capture function
    |     LastModbusFunction = ModbusFunction;
    | end
  function readModbusResponse:
    | function readModbusResponse %#codegen
    |     % Insert the new data into the SerialBuffer
    |     numNewBytes = min(SerialIn(1), 256);
    |     assert(numNewBytes < 257);
    |     SerialBuffer(SerialBufferEnd + (1:numNewBytes)) = SerialIn(1 + (1:numNewBytes));
    |     SerialBufferEnd = SerialBufferEnd + numNewBytes;
    |     
    |     Valid = false; % Invalid packet
    |     if (SerialBuffer(2) == LastModbusFunction) && (SerialBufferEnd == 3 + ResponseLength)
    |         Valid = true; % Okay
    |     elseif (SerialBuffer(2) == LastModbusFunction+128) && (SerialBufferEnd == 5)
    |         Valid = true; % Exception
    |     end
    | 
    | end
  function sendStreamingCmd(Select):
    | function sendStreamingCmd(Select) %#codegen
    |     
    |     Function = uint16(70);
    |     if (Select==1)
    |         L = 2;
    |         Data = 85;
    |     else
    |         L = 16;
    |         Data = 85*ones(L-1,1,'uint32'); % JAMMING SEQUENCE
    |     end
    |     sendModbusCmd(uint32([L; Function; Data])) %#codegen
    | end
  function validateModbusResponse:
    | function validateModbusResponse %#codegen
    |     Valid = false;
    |     ModbusResponse = zeros(256, 1, 'uint32');
    |     
    |     if (SerialBuffer(2) == LastModbusFunction) && (SerialBufferEnd == 3 + ResponseLength) ...
    |             || (SerialBuffer(2) == LastModbusFunction + 128) && (SerialBufferEnd == 5)
    |         
    |         Valid = checkModbusCRC32(SerialBuffer(1:SerialBufferEnd));
    |         if Valid
    |             % Strip off the Modbus Address and CRC
    |             L = SerialBufferEnd-3;
    |             assert(L < 255);
    |             ModbusResponse(1) = uint32(L);
    |             ModbusResponse(1+(1:L)) = SerialBuffer(1+(1:L));
    |         end
    |     end
    | end
  function clearModbusCommand:
    | function clearModbusCommand %#codegen
    |     ModbusCommand = zeros(65, 1, 'uint32');
    | end
  function clearCalibration:
    | function clearCalibration %#codegen
    |     Calibration       = FTCalibration;
    |     CalibrationBuffer = zeros(512, 1, 'uint32');
    |     CalibrationBufferEnd = uint32(0);
    | end
  function clearSerialOut:
    | function clearSerialOut %#codegen
    |     SerialOut = zeros(65, 1, 'uint32');
    | end
  function clearModbusResponse:
    | function clearModbusResponse %#codegen
    |     ModbusResponse(1) = uint32(0);
    |     ModbusStatus = 0;
    | end
  function clearSerialBuffer:
    | function clearSerialBuffer %#codegen
    |     SerialBuffer = zeros(512, 1, 'uint32');
    |     SerialBufferEnd = uint32(0);
    | end
  function clearGauge:
    | function clearGauge %#codegen
    |     Gauge = zeros(6,1);
    |     GaugeStatus = 0;
    | end
